simulink model "continous_observer"  (R2020b)
settings: Solver=VariableStepAuto  StartTime=0.0  StopTime=100  RelTol=1e-3
values from neighbouring files (symbols this model uses):
  A = [0 -theta2 0; 0 -1/theta3 1/theta3; 0 0 -1/theta3]    [script1.m]
  B = [0; 0; 1/theta3]    [script1.m]
  C = [1 0 0]    [script1.m]
  F_k = k*[1/theta2 -theta3 -theta3]    [script1.m]
undefined symbols (not defined in the file or in its folder): L
settings Model: Creator=Francesco  LastModifiedBy=Francesco

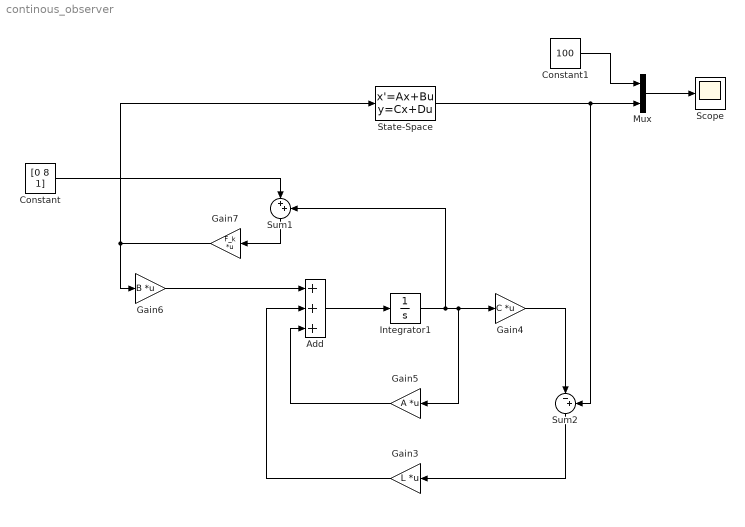
== system continous_observer ==
  Add : Sum  Inputs=+++
  Constant : Constant  Value=[0 8 1]
  Constant1 : Constant  Value=100
  Gain3 : Gain  Gain=L  Multiplication=Matrix(K*u)
  Gain4 : Gain  Gain=C  Multiplication=Matrix(K*u)
  Gain5 : Gain  Gain=A  Multiplication=Matrix(K*u)
  Gain6 : Gain  Gain=B  Multiplication=Matrix(K*u)
  Gain7 : Gain  Gain=F_k  Multiplication=Matrix(K*u)
  Integrator1 : Integrator
  Mux : Mux  Inputs=2
  Scope : Scope
  State-Space : StateSpace  A=A  B=B  C=C  D=0  InitialCondition=[337 192 0]
  Sum1 : Sum  Inputs=|++
  Sum2 : Sum  Inputs=|-+
  wires:
  Integrator1/1 -> Gain5/1, Gain4/1, Sum1/2
  Add/1 -> Integrator1/1
  Gain5/1 -> Add/3
  Gain3/1 -> Add/2
  Gain4/1 -> Sum2/1
  State-Space/1 -> Mux/2, Sum2/2
  Sum2/1 -> Gain3/1
  Gain6/1 -> Add/1
  Sum1/1 -> Gain7/1
  Constant/1 -> Sum1/1
  Gain7/1 -> State-Space/1, Gain6/1
  Constant1/1 -> Mux/1
  Mux/1 -> Scope/1
